simulink model "interfaceTemplate"  (Simulink 7.6)
settings: Solver=ode45  StartTime=0.0  StopTime=10.0  RelTol=1e-3
settings Model: Creator=chepeadan  LastModifiedBy=chepeadan
settings DebuggingCC: StrictBusMsg=Warning

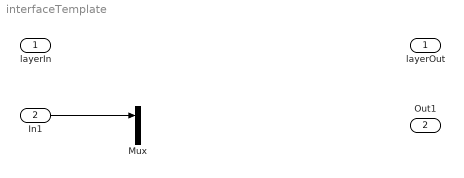
== system interfaceTemplate ==
  layerIn : Inport
  In1 : Inport  Port=2
  Mux : Mux  Inputs=2
  layerOut : Outport
  Out1 : Outport  Port=2
  wires:
  In1/1 -> Mux/1
